simulink model "balance_lqr"  (R2022a)
settings: Solver=VariableStepAuto  StartTime=0.0  StopTime=20  RelTol=1e-3
undefined symbols (not defined in the file): A1, A2, B1, B2, B3, K11, K12, K13, K14, K15, K16, K21, K22, K23, K24, K25, K26, v
settings Model: Creator=HXZP  LastModifiedBy=HXZP

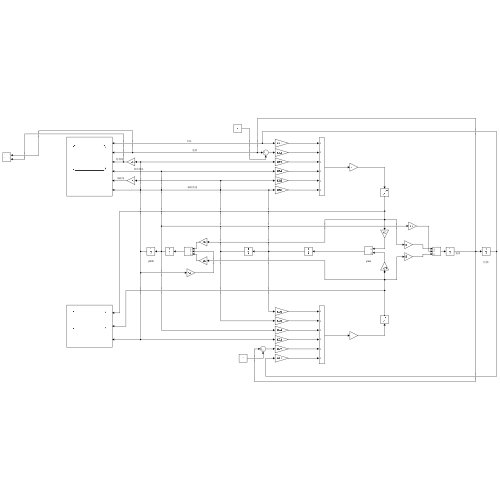
[thumbnail: Simulink's stored preview of the top-level diagram]
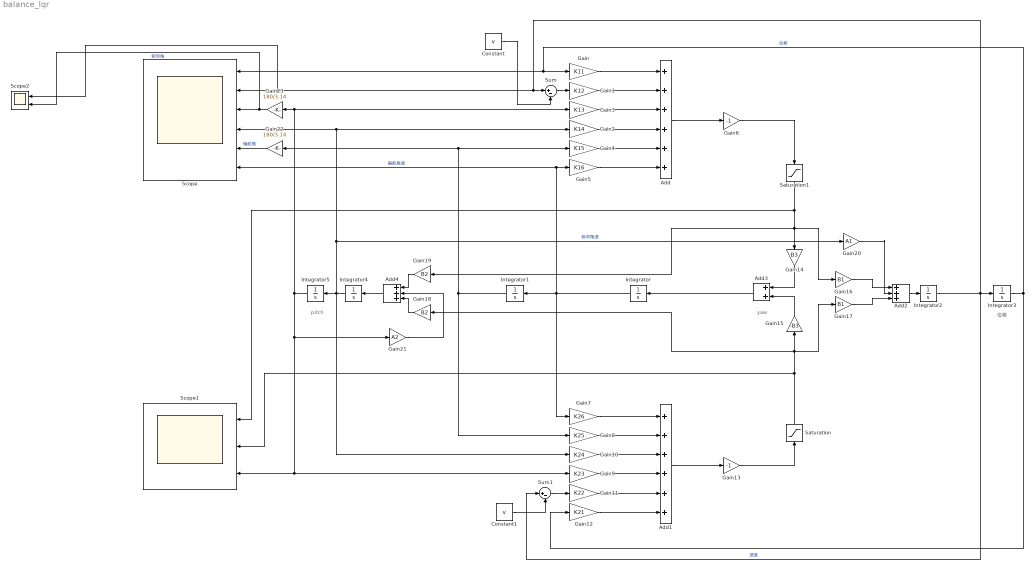
== system balance_lqr ==
  note: yaw
  note: 位移
  note: pitch
  Add : Sum  Inputs=++++++
  Add1 : Sum  Inputs=++++++
  Add2 : Sum  Inputs=+++
  Add3 : Sum
  Add4 : Sum  Inputs=+++
  Constant : Constant  Value=v
  Constant1 : Constant  Value=v
  Gain : Gain  Gain=K11
  Gain1 : Gain  Gain=K12
  Gain10 : Gain  Gain=K24
  Gain11 : Gain  Gain=K22
  Gain12 : Gain  Gain=K21
  Gain13 : Gain  Gain=-1
  Gain14 : Gain  Gain=B3
  Gain15 : Gain  Gain=-B3
  Gain16 : Gain  Gain=B1
  Gain17 : Gain  Gain=B1
  Gain18 : Gain  Gain=B2
  Gain19 : Gain  Gain=B2
  Gain2 : Gain  Gain=K14
  Gain20 : Gain  Gain=A1
  Gain21 : Gain  Gain=A2
  Gain22 : Gain  Gain=180/3.14
  Gain23 : Gain  Gain=180/3.14
  Gain3 : Gain  Gain=K13
  Gain4 : Gain  Gain=K15
  Gain5 : Gain  Gain=K16
  Gain6 : Gain  Gain=-1
  Gain7 : Gain  Gain=K26
  Gain8 : Gain  Gain=K25
  Gain9 : Gain  Gain=K23
  Integrator{,1..5} (6 alike) : Integrator
  Saturation : Saturate  UpperLimit=5  LowerLimit=-5
  Saturation1 : Saturate  UpperLimit=5  LowerLimit=-5
  Scope : Scope  NumInputPorts=6
  Scope1 : Scope  NumInputPorts=3
  Scope2 : Scope  NumInputPorts=2
  Sum : Sum  Inputs=|+-
  Sum1 : Sum  Inputs=|+-
  wires:
  Gain/1 -> Add/1
  Gain1/1 -> Add/2
  Gain3/1 -> Add/3
  Gain2/1 -> Add/4
  Gain4/1 -> Add/5
  Gain5/1 -> Add/6
  Add/1 -> Gain6/1
  Gain12/1 -> Add1/6
  Gain8/1 -> Add1/2
  Gain9/1 -> Add1/4
  Gain7/1 -> Add1/1
  Add1/1 -> Gain13/1
  Gain11/1 -> Add1/5
  Gain10/1 -> Add1/3
  Gain15/1 -> Add3/2
  Gain14/1 -> Add3/1
  Add3/1 -> Integrator/1
  Integrator/1 -> Scope/6, Gain5/1, Gain7/1, Integrator1/1  "偏航角速"
  Integrator1/1 -> Gain8/1, Gain4/1, Gain22/1
  Gain16/1 -> Add2/1
  Add2/1 -> Integrator2/1
  Integrator2/1 -> Sum1/1, Sum/1, Scope2/1, Scope/2, Integrator3/1  "速度"
  Integrator3/1 -> Gain/1, Scope/1, Gain12/1  "位移"
  Gain17/1 -> Add2/3
  Gain19/1 -> Add4/1
  Gain18/1 -> Add4/3
  Add4/1 -> Integrator4/1
  Integrator4/1 -> Scope/4, Gain2/1, Gain20/1, Gain10/1, Integrator5/1  "俯仰角速"
  Integrator5/1 -> Gain9/1, Scope1/3, Gain21/1, Gain3/1, Gain23/1
  Gain20/1 -> Add2/2
  Gain21/1 -> Add4/2
  Gain23/1 -> Scope2/2, Scope/3  "俯仰角"
  Gain22/1 -> Scope/5  "偏航角"
  Gain6/1 -> Saturation1/1
  Gain13/1 -> Saturation/1
  Sum/1 -> Gain1/1
  Constant/1 -> Sum/2
  Sum1/1 -> Gain11/1
  Constant1/1 -> Sum1/2
  Saturation/1 -> Gain18/1, Gain17/1, Gain15/1, Scope1/2
  Saturation1/1 -> Gain14/1, Gain19/1, Gain16/1, Scope1/1
